simulink model "AutonomousControl"  (R2015a)
settings: Solver=ode45  StartTime=0.0  StopTime=inf  FixedStep=0.01  RelTol=1e-3
libraries: simulink x11, dspindex x8, dspnetwork x3, aerolibconvert2 x1, IMU_Library x1, GPS_Library x1, realtime_pacer_lib x1, etargetslib x1
(part 2 of 2)

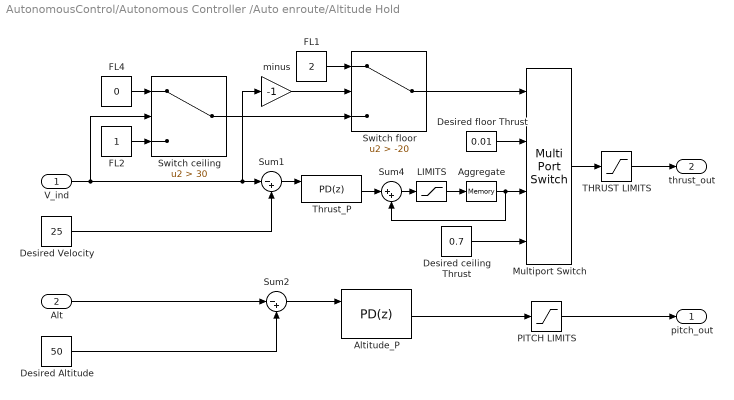
== system AutonomousControl/Autonomous Controller /Auto enroute/Altitude Hold ==
  V_ind : Inport
  Alt : Inport  Port=2
  Aggregate : Memory
  Altitude_P : simulink/Continuous/PID Controller  Controller=PD  TimeDomain=Discrete-time  SampleTime=0.02  IntegratorMethod=Forward Euler  FilterMethod=Forward Euler  Form=Parallel  UseFilter=off  ControllerParametersSource=internal  P=0.12  I=0.0003  D=0.0024  N=20  InitialConditionSource=internal  InitialConditionForIntegrator=0  InitialConditionForFilter=0  ExternalReset=either  LimitOutput=on  UpperSaturationLimit=1  LowerSaturationLimit=-1  LinearizeAsGain=on  AntiWindupMode=none  Kb=1  TrackingMode=off  Kt=1  PParamMin=[]  PParamMax=[]  IParamMin=[]  IParamMax=[]  DParamMin=[]  DParamMax=[]  NParamMin=[]  NParamMax=[]  KbParamMin=[]  KbParamMax=[]  KtParamMin=[]  KtParamMax=[]  POutMin=[]  POutMax=[]  IOutMin=[]  IOutMax=[]  DOutMin=[]  DOutMax=[]  NOutMin=[]  NOutMax=[]  KbOutMin=[]  KbOutMax=[]  KtOutMin=[]  KtOutMax=[]  IntegratorOutMin=[]  IntegratorOutMax=[]  FilterOutMin=[]  FilterOutMax=[]  SumOutMin=[]  SumOutMax=[]  SumI1OutMin=[]  SumI1OutMax=[]  SumI2OutMin=[]  SumI2OutMax=[]  SumI3OutMin=[]  SumI3OutMax=[]  SumDOutMin=[]  SumDOutMax=[]  SaturationOutMin=[]  SaturationOutMax=[]  IntegratorContinuousStateAttributes=''  IntegratorStateMustResolveToSignalObject=off  IntegratorRTWStateStorageClass=Auto  FilterContinuousStateAttributes=''  FilterStateMustResolveToSignalObject=off  FilterRTWStateStorageClass=Auto  DifferentiatorICPrevScaledInput=0  DifferentiatorOutMin=[]  DifferentiatorOutMax=[]
  Desired Altitude : Constant  Value=50  OutDataTypeStr=single
  Desired Velocity : Constant  Value=25  OutDataTypeStr=single
  "Desired ceiling Thrust " : Constant  Value=0.7  OutDataTypeStr=single
  Desired floor Thrust : Constant  Value=0.01  OutDataTypeStr=single
  FL1 : Constant  Value=2  OutDataTypeStr=single
  FL2 : Constant  OutDataTypeStr=single
  FL4 : Constant  Value=0  OutDataTypeStr=single
  LIMITS : Saturate  UpperLimit=0.4  LowerLimit=0
  Multiport Switch : MultiPortSwitch  DataPortOrder=Zero-based contiguous
  PITCH LIMITS : Saturate  UpperLimit=0.4  LowerLimit=-0.4
  Sum1 : Sum  Inputs=|-+
  Sum2 : Sum  Inputs=|-+
  Sum4 : Sum  Inputs=|++
  Switch ceiling : Switch  Criteria=u2 > Threshold  Threshold=30
  Switch floor : Switch  Criteria=u2 > Threshold  Threshold=-20
  THRUST LIMITS : Saturate  UpperLimit=1  LowerLimit=0
  Thrust_P : simulink/Continuous/PID Controller  Controller=PD  TimeDomain=Discrete-time  SampleTime=0.02  IntegratorMethod=Forward Euler  FilterMethod=Forward Euler  Form=Parallel  UseFilter=off  ControllerParametersSource=internal  P=0.0005  I=0.0000000001  D=0.003  N=20  InitialConditionSource=internal  InitialConditionForIntegrator=0  InitialConditionForFilter=0  ExternalReset=either  LimitOutput=on  UpperSaturationLimit=1  LowerSaturationLimit=-1  LinearizeAsGain=on  AntiWindupMode=none  Kb=1  TrackingMode=off  Kt=1  PParamMin=[]  PParamMax=[]  IParamMin=[]  IParamMax=[]  DParamMin=[]  DParamMax=[]  NParamMin=[]  NParamMax=[]  KbParamMin=[]  KbParamMax=[]  KtParamMin=[]  KtParamMax=[]  POutMin=[]  POutMax=[]  IOutMin=[]  IOutMax=[]  DOutMin=[]  DOutMax=[]  NOutMin=[]  NOutMax=[]  KbOutMin=[]  KbOutMax=[]  KtOutMin=[]  KtOutMax=[]  IntegratorOutMin=[]  IntegratorOutMax=[]  FilterOutMin=[]  FilterOutMax=[]  SumOutMin=[]  SumOutMax=[]  SumI1OutMin=[]  SumI1OutMax=[]  SumI2OutMin=[]  SumI2OutMax=[]  SumI3OutMin=[]  SumI3OutMax=[]  SumDOutMin=[]  SumDOutMax=[]  SaturationOutMin=[]  SaturationOutMax=[]  IntegratorContinuousStateAttributes=''  IntegratorStateMustResolveToSignalObject=off  IntegratorRTWStateStorageClass=Auto  FilterContinuousStateAttributes=''  FilterStateMustResolveToSignalObject=off  FilterRTWStateStorageClass=Auto  DifferentiatorICPrevScaledInput=0  DifferentiatorOutMin=[]  DifferentiatorOutMax=[]
  minus : Gain  Gain=-1
  pitch_out : Outport
  thrust_out : Outport  Port=2
  wires:
  PITCH LIMITS/1 -> pitch_out/1
  Sum2/1 -> Altitude_P/1
  Desired Altitude/1 -> Sum2/2
  Altitude_P/1 -> PITCH LIMITS/1
  Sum1/1 -> Thrust_P/1
  Desired Velocity/1 -> Sum1/2
  Sum4/1 -> LIMITS/1
  Thrust_P/1 -> Sum4/1
  Alt/1 -> Sum2/1
  Switch ceiling/1 -> Switch floor/3
  V_ind/1 -> Switch ceiling/2, minus/1, Sum1/1
  minus/1 -> Switch floor/2
  Switch floor/1 -> Multiport Switch/1
  FL1/1 -> Switch floor/1
  Desired floor Thrust/1 -> Multiport Switch/2
  Multiport Switch/1 -> THRUST LIMITS/1
  FL4/1 -> Switch ceiling/1
  FL2/1 -> Switch ceiling/3
  "Desired ceiling Thrust "/1 -> Multiport Switch/4
  THRUST LIMITS/1 -> thrust_out/1
  LIMITS/1 -> Aggregate/1
  Aggregate/1 -> Multiport Switch/3, Sum4/2

== system AutonomousControl/Autonomous Controller /Auto Landing/On-track indicator/one-way switch  ==
  In : Inport
  Memory4 : Memory  InheritSampleTime=on
  Switch8 : Switch  Criteria=u2 > Threshold
  Out : Outport
  wires:
  Memory4/1 -> Out/1, Switch8/3
  Switch8/1 -> Memory4/1
  In/1 -> Switch8/1, Switch8/2

== system AutonomousControl/Autonomous Controller /Auto Take-off/Enroute Indicator/one-way switch  ==
  In : Inport
  Memory4 : Memory  InheritSampleTime=on
  Switch8 : Switch  Criteria=u2 > Threshold
  Out : Outport
  wires:
  Memory4/1 -> Out/1, Switch8/3
  Switch8/1 -> Memory4/1
  In/1 -> Switch8/1, Switch8/2

== system AutonomousControl/Autonomous Controller /Auto Take-off/Velocity Indicator/one-way switch  ==
  In : Inport
  Memory4 : Memory  InheritSampleTime=on
  Switch8 : Switch  Criteria=u2 > Threshold
  Out : Outport
  wires:
  Memory4/1 -> Out/1, Switch8/3
  Switch8/1 -> Memory4/1
  In/1 -> Switch8/1, Switch8/2

== matlab function AutonomousControl/Send to XPlane10/'DATA0' ==
  data: y output
function y = fcn()
%#codegen
%y=uint8(zeros(1,77));
y = uint8('DATA0');

== matlab function AutonomousControl/Get data from XPlane/MATLAB Function ==
  data: u input; Data output single size=[30 8]; msgLen input
function Data  = fcn(u,msgLen)
%#codegen
%coder.extrinsic('clear')
dataLen=msgLen-5;
Npackets=dataLen/36;

% initialize data matrix
% rows: packets of data; columns: data values, first column is the data
% index
maxNPackets=30;
Nvalues=8;% number of values in each packet
Data=single(zeros(maxNPackets,Nvalues));

Bytecounter=6; % start after the 5th byte

for i=1:msgLen
    
    if char(u(i))=='D' && char(u(i+1))=='A'
        %loop over each packet
        for j=1:Npackets
                indx=typecast(u(Bytecounter:Bytecounter+3),'uint32');% packet index
                %Data(indx,1)=single(indx); % packet index
                Bytecounter=Bytecounter+4; % go to the next 4 bytes
                Data(indx,1)=typecast(u(Bytecounter:Bytecounter+3),'single'); % 1st value
                Bytecounter=Bytecounter+4; % go to the next 4 bytes
                Data(indx,2)=typecast(u(Bytecounter:Bytecounter+3),'single'); % 2nd value
                Bytecounter=Bytecounter+4; % go to the next 4 bytes
                Data(indx,3)=typecast(u(Bytecounter:Bytecounter+3),'single'); % 3rd value
                Bytecounter=Bytecounter+4; % go to the next 4 bytes
                Data(indx,4)=typecast(u(Bytecounter:Bytecounter+3),'single'); % 4th value
                Bytecounter=Bytecounter+4; % go to the next 4 bytes
                Data(indx,5)=typecast(u(Bytecounter:Bytecounter+3),'single'); % 5th value
                Bytecounter=Bytecounter+4; % go to the next 4 bytes
                Data(indx,6)=typecast(u(Bytecounter:Bytecounter+3),'single'); % 6th value
                Bytecounter=Bytecounter+4; % go to the next 4 bytes
                Data(indx,7)=typecast(u(Bytecounter:Bytecounter+3),'single'); % 7th value
                Bytecounter=Bytecounter+4; % go to the next 4 bytes
                Data(indx,8)=typecast(u(Bytecounter:Bytecounter+3),'single'); % 8th value
                Bytecounter=Bytecounter+4;% go to the next packet index 
        end
        break
    end
end
%clear Data

== matlab function AutonomousControl/Autonomous Controller /Auto enroute/MATLAB Function2 ==
  data: currentPosition input; WP input; targetHeading output; status output
function [targetHeading, status] = azimuthCal(currentPosition, WP)
%=============================Intitialization==============================
persistent initialize index sizeWPArray currentWP stt;
    
if isempty(initialize)
    if isempty(index)
        index = 1;  
        currentWP = [0 0 0];
        stt = 0;
    end    
    sizeWPArray = length(WP(:,1));  
    initialize = 1;
else
    if(norm(-transpose(currentPosition(1:2)) + WP(index,1:2)) < 5e-04)
        if (index < sizeWPArray)
            index = index + 1;      
        else
            stt = 1;
        end
    end     
end

currentWP = WP(index,:);
status = stt;
%Declare azimuth as extrinsic
coder.extrinsic('azimuth'); 
targetHeading = coder.nullcopy(zeros(1));
targetHeading = azimuth(currentPosition(1),currentPosition(2),currentWP(1),currentWP(2));

== matlab function AutonomousControl/MATLAB Function1 ==
  data: AirportCoordinates output
function AirportCoordinates = getWP()
AirportCoordinates = [21.219041824340820 105.8135528564453 50; 21.225227355957030 105.7927398681641 50];
% AirportCoordinates = [21.219041824340820 105.8135528564453 50; 21.221620559692383 1.058050003051758e+02 50; 21.225227355957030 105.7927398681641 50];
% WPdataTable = [21.215 105.798 50; 21.219041824340820 105.8135528564453 50; 21.225227355957030 105.7927398681641 50];
% 21.220420837402344 1.058090286254883e+02;
% 21.221620559692383 1.058050003051758e+02;

== matlab function AutonomousControl/MATLAB Function2 ==
  data: WPdataTable output
function WPdataTable = getWP()
WPdataTable = [21.215 105.798 50; 21.219041824340820 105.8135528564453 50];
% WPdataTable = [21.215 105.798 50; 21.219041824340820 105.8135528564453 50; 21.225227355957030 105.7927398681641 50];
% 21.220420837402344 1.058090286254883e+02;
% 21.221620559692383 1.058050003051758e+02;

== matlab function AutonomousControl/Autonomous Controller /Auto Landing/MATLAB Function2 ==
  data: currentPosition input; WP input; ref_azimuth output; curr_azimuth output
function [ref_azimuth, curr_azimuth] = currentWP(currentPosition, WP)
%=============================Intitialization==============================
persistent initialize curr_buff;
    
if isempty(initialize)
    if isempty(curr_buff)        
        curr_buff = coder.nullcopy(zeros(1));
        ref_azimuth = coder.nullcopy(zeros(1));
    end        
    initialize = 1;     
end
%Declare patch as extrinsic
coder.extrinsic('azimuth'); 
curr_buff = azimuth(currentPosition(1),currentPosition(2),WP(2,1),WP(2,2));
ref_azimuth = azimuth(WP(1,1),WP(1,2),WP(2,1),WP(2,2));
curr_azimuth = curr_buff;
